simulink model "Sim_moteur2"  (R2023a)
settings: Solver=FixedStepAuto  StartTime=0.0  StopTime=3  FixedStep=1e-5  RelTol=1e-3
values from neighbouring files (symbols this model uses):
  Cr = 0    [main.m]    (also in main2.m; main3.m; matlab.mat)
  f = 1.52e-4    (= 0.000152)    [main.m]    (also in main2.m; main3.m; matlab.mat)
  g_annule = 1/(-C_etat*inv(A_etat-B_etat*Kt)*B_etat)    [main2.m]    (also in main3.m; matlab.mat = 1992.67173058)
  Jtot = Jmot+m*(pas/(2*pi))^2    (= 4.78232346171e-05)    [main.m]    (also in main2.m; main3.m; matlab.mat)
  Ka = 0.1    [main.m]    (also in main2.m; main3.m; matlab.mat)
  Kc = 5.7e-2    (= 0.057)    [main.m]    (also in main2.m; main3.m; matlab.mat)
  Kr = K_ac(3)    [main2.m]    (also in main3.m; matlab.mat = -2846.67390083)
  Kt = [K1, K2]    [main2.m]    (also in main3.m; matlab.mat = [1992.67173058 434854.47797])
  pas = 5e-3    (= 0.005)    [main.m]    (also in main2.m; main3.m; matlab.mat)
settings Model: Creator=philippecasteres  LastModifiedBy=philippecasteres

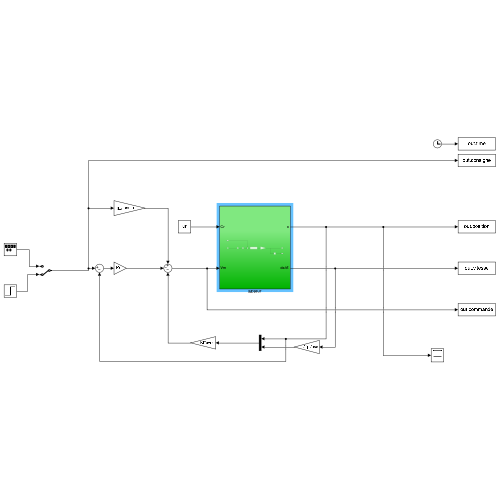
[thumbnail: Simulink's stored preview of the top-level diagram]
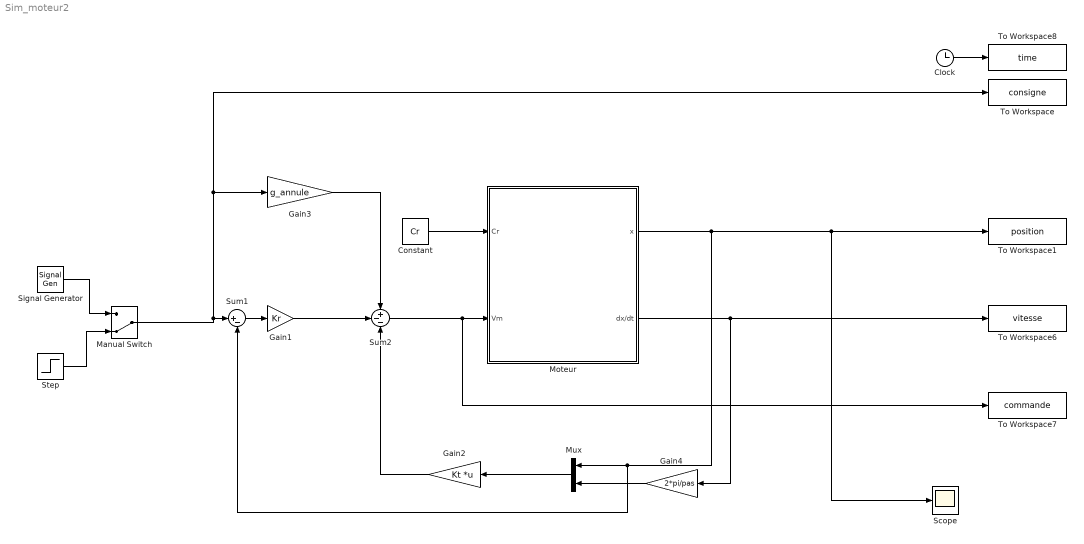
== system Sim_moteur2 ==
  Clock : Clock
  Constant : Constant  Value=Cr
  Gain1 : Gain  Gain=Kr
  Gain2 : Gain  Gain=Kt  Multiplication=Matrix(K*u) (u vector)
  Gain3 : Gain  Gain=g_annule
  Gain4 : Gain  Gain=2*pi/pas
  Manual Switch : ManualSwitch  CurrentSetting=0
  Moteur : Subsystem
  Mux : Mux  Inputs=2
  Scope : Scope
  Signal Generator : SignalGenerator  WaveForm=square  Amplitude=0.35  Frequency=0.5  Units=rad/sec
  Step : Step  Time=0  After=0.35  SampleTime=0
  Sum1 : Sum  Inputs=|+-
  Sum2 : Sum  Inputs=+--
  To Workspace : ToWorkspace  VariableName=consigne  SaveFormat=Timeseries  SampleTime=-1
  To Workspace1 : ToWorkspace  VariableName=position  SaveFormat=Timeseries  SampleTime=-1
  To Workspace6 : ToWorkspace  VariableName=vitesse  SaveFormat=Timeseries  SampleTime=-1
  To Workspace7 : ToWorkspace  VariableName=commande  SaveFormat=Timeseries  SampleTime=-1
  To Workspace8 : ToWorkspace  VariableName=time  SaveFormat=Timeseries  SampleTime=-1
  wires:
  Moteur/2(dx/dt) -> Gain4/1, To Workspace6/1
  Signal Generator/1 -> Manual Switch/1
  Step/1 -> Manual Switch/2
  Constant/1 -> Moteur/1(Cr)
  Gain1/1 -> Sum2/2
  Clock/1 -> To Workspace8/1
  Manual Switch/1 -> Sum1/1, To Workspace/1, Gain3/1
  Sum2/1 -> To Workspace7/1, Moteur/2(Vm)
  Sum1/1 -> Gain1/1
  Mux/1 -> Gain2/1
  Gain2/1 -> Sum2/3
  Gain3/1 -> Sum2/1
  Moteur/1(x) -> Sum1/2, Mux/1, Scope/1, To Workspace1/1
  Gain4/1 -> Mux/2

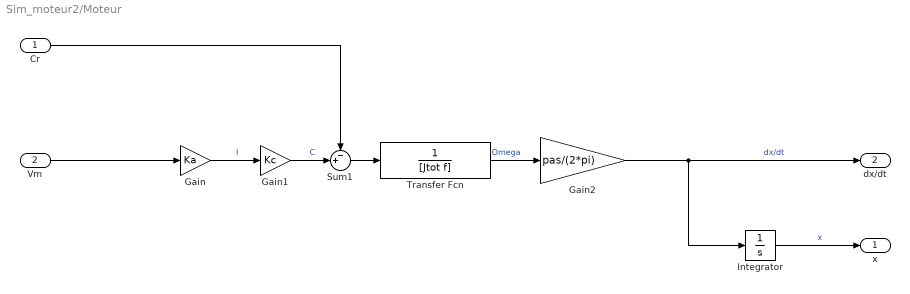
== system Sim_moteur2/Moteur ==
  Cr : Inport
  Vm : Inport  Port=2
  Gain : Gain  Gain=Ka
  Gain1 : Gain  Gain=Kc
  Gain2 : Gain  Gain=pas/(2*pi)
  Integrator : Integrator
  Sum1 : Sum  Inputs=-+|
  Transfer Fcn : TransferFcn  Denominator=[Jtot f]
  x : Outport
  dx/dt : Outport  Port=2
  wires:
  Cr/1 -> Sum1/1
  Vm/1 -> Gain/1
  Gain/1 -> Gain1/1  "I"
  Integrator/1 -> x/1  "x"
  Sum1/1 -> Transfer Fcn/1
  Gain1/1 -> Sum1/2  "C"
  Gain2/1 -> dx/dt/1, Integrator/1  "dx/dt"
  Transfer Fcn/1 -> Gain2/1  "Omega"
